simulink model "Prob2_MBD"  (R2020b)
settings: Solver=VariableStepAuto  StartTime=0.0  StopTime=100.0  RelTol=1e-3
InitFcn:
  | M1=5000;
  | k1=50;
  | b=50;
  | k2=10000;
  | M2=100;
settings Model: Creator=Ani  LastModifiedBy=Ani

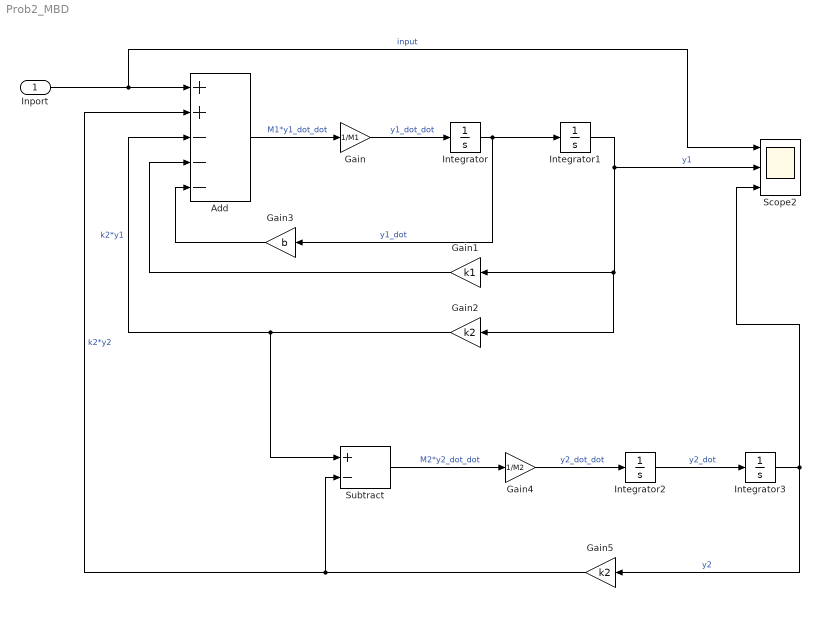
== system Prob2_MBD ==
  Inport : Inport
  Add : Sum  Inputs=++---
  Gain : Gain  Gain=1/M1
  Gain1 : Gain  Gain=k1
  Gain2 : Gain  Gain=k2
  Gain3 : Gain  Gain=b
  Gain4 : Gain  Gain=1/M2
  Gain5 : Gain  Gain=k2
  Integrator{,1..3} (4 alike) : Integrator
  Scope2 : Scope  NumInputPorts=3
      settings: InitFcn=|
      | M1=5000;
      | k1=50;
      | b=50;
      | k2=10000;
      | M2=100
  Subtract : Sum  Inputs=+-
  wires:
  Inport/1 -> Scope2/1, Add/1  "input"
  Integrator3/1 -> Scope2/3, Gain5/1  "y2"
  Integrator1/1 -> Gain2/1, Gain1/1, Scope2/2  "y1"
  Gain3/1 -> Add/5
  Gain/1 -> Integrator/1  "y1_dot_dot"
  Gain2/1 -> Subtract/1, Add/3  "k2*y1"
  Gain5/1 -> Add/2, Subtract/2  "k2*y2"
  Subtract/1 -> Gain4/1  "M2*y2_dot_dot"
  Gain4/1 -> Integrator2/1  "y2_dot_dot"
  Add/1 -> Gain/1  "M1*y1_dot_dot"
  Gain1/1 -> Add/4
  Integrator/1 -> Gain3/1, Integrator1/1  "y1_dot"
  Integrator2/1 -> Integrator3/1  "y2_dot"
